simulink model "Problem2"  (R2020b)
settings: Solver=VariableStepAuto  StartTime=0.0  StopTime=10.0  RelTol=1e-3
values from neighbouring files (symbols this model uses):
  b = 290    [Parameters.m]
  M1 = 465    [Parameters.m]
  M2 = 50    [Parameters.m]
undefined symbols (not defined in the file or in its folder): k1, k2
settings Model: Creator=adity  LastModifiedBy=adity

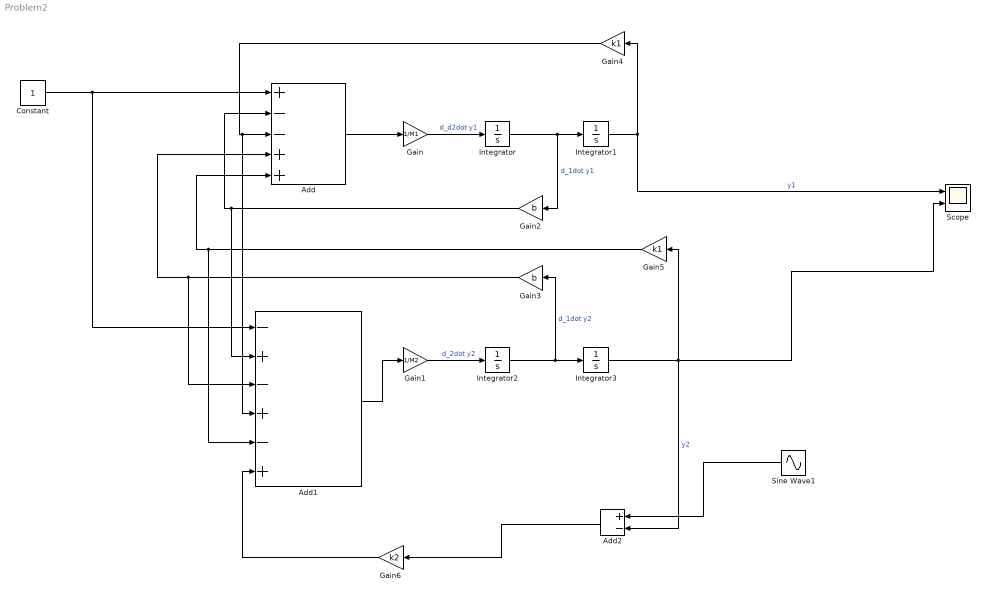
== system Problem2 ==
  Add : Sum  Inputs=+--++
  Add1 : Sum  Inputs=-+-+-+
  Add2 : Sum  Inputs=+-
  Constant : Constant
  Gain : Gain  Gain=1/M1
  Gain1 : Gain  Gain=1/M2
  Gain2 : Gain  Gain=b
  Gain3 : Gain  Gain=b
  Gain4 : Gain  Gain=k1
  Gain5 : Gain  Gain=k1
  Gain6 : Gain  Gain=k2
  Integrator{,1..3} (4 alike) : Integrator
  Scope : Scope  NumInputPorts=2
  Sine Wave1 : Sin  Amplitude=2  Frequency=10  SampleTime=0
  wires:
  Add1/1 -> Gain1/1
  Add2/1 -> Gain6/1
  Gain3/1 -> Add1/3, Add/4
  Add/1 -> Gain/1
  Gain4/1 -> Add1/4, Add/3
  Gain1/1 -> Integrator2/1  "d_2dot y2"
  Integrator2/1 -> Gain3/1, Integrator3/1  "d_1dot y2"
  Sine Wave1/1 -> Add2/1
  Gain2/1 -> Add1/2, Add/2
  Constant/1 -> Add/1, Add1/1
  Gain6/1 -> Add1/6
  Integrator1/1 -> Gain4/1, Scope/1  "y1"
  Integrator/1 -> Gain2/1, Integrator1/1  "d_1dot y1"
  Integrator3/1 -> Add2/2, Scope/2, Gain5/1  "y2"
  Gain5/1 -> Add1/5, Add/5
  Gain/1 -> Integrator/1  "d_d2dot y1"
